simulink model "GS_model"  (R2018b)
settings: Solver=ode5  StartTime=0.0  StopTime=SimuStopTime  FixedStep=T_Simu  RelTol=1e-3
InitFcn:
  | Initial
undefined symbols (not defined in the file or in its folder): Aba10, Aba20, aeroCIP2006_S, aeroCIP2006_X, aeroCIP2006_Y, Agl0, Ass_kS, Ass_n1, Ass_n2, Ass_n3, Ass_n4, Ass_Noise, Ass_R, Ass_Resolution, Ass_TmOrder, AssA_Fix_Abs, AssB_Fix_Abs, AssC_Fix_Abs, AssD_Fix_Abs, AssE_Fix_Aps, AssF_Fix_Aps, C, c_max, c_min, Cd, CenterOfFigNX, CenterOfFigNY, CenterOfFigNZ, CenterOfFigP1, CenterOfFigP2, CenterOfFigPX, CenterOfFigPY, CenterOfFigPZ, Cmu, Crou, DEG2RAD, DiscIntNeverNeededParam, Eg_Dir, Eg_F, Eg_PrepareTime, Eg_r_L_L, Fw_Abf, Fw_Hmax, Fw_J, Fw_Spd0, Fw_Tmax, git_hash_BaseLine, git_hash_Project, Gnss_Noise_Pos, Gnss_Noise_Vel, Gnss_PropgationTime, GyroA_Fix_Abg, GyroA_Noise, GyroB_Fix_Abg, GyroB_Noise, GyroC_Fix_Abg, GyroC_Noise, GyroD_Fix_Abg, GyroD_Noise, h ... (+94)
libraries: simulink x308, sharedutil x46, aerolibutil x37, sharedtransform x31, vrlib x14, aerolibgravity2 x2
(part 16 of 20)

== system GS_model/Subsystem2/Subsystem/Sensor/Magnetometer/MmModel2/Mm_ErrSet/MmErrSet/MmErrSet_Wave ==
  Mm_in : Inport
  ErrSet : Inport  Port=2
  Constant1 : Constant  Value=2
  Constant2 : Constant  Value=3
  Constant3 : Constant
  Demux : Demux  Outputs=3
  MmAxisXErrSet_Wave : Subsystem
  MmAxisXErrSet_Wave1 : Subsystem
  MmAxisXErrSet_Wave2 : Subsystem
  Mux : Mux  Inputs=3
  WaveSet : SignalGenerator  WaveForm=square  Amplitude=0.2
  Mm_out : Outport
  wires:
  Demux/3 -> MmAxisXErrSet_Wave2/1(MmAxis_in)
  Demux/2 -> MmAxisXErrSet_Wave1/1(MmAxis_in)
  Constant2/1 -> MmAxisXErrSet_Wave2/3(MmAxis_Num)
  Constant1/1 -> MmAxisXErrSet_Wave1/3(MmAxis_Num)
  MmAxisXErrSet_Wave2/1(MmAxis_out) -> Mux/3
  MmAxisXErrSet_Wave/1(MmAxis_out) -> Mux/1
  MmAxisXErrSet_Wave1/1(MmAxis_out) -> Mux/2
  WaveSet/1 -> MmAxisXErrSet_Wave/4(MmAxis_WaveSet), MmAxisXErrSet_Wave1/4(MmAxis_WaveSet), MmAxisXErrSet_Wave2/4(MmAxis_WaveSet)
  Constant3/1 -> MmAxisXErrSet_Wave/3(MmAxis_Num)
  ErrSet/1 -> MmAxisXErrSet_Wave/2(ErrSet), MmAxisXErrSet_Wave1/2(ErrSet), MmAxisXErrSet_Wave2/2(ErrSet)
  Demux/1 -> MmAxisXErrSet_Wave/1(MmAxis_in)
  Mux/1 -> Mm_out/1
  Mm_in/1 -> Demux/1

== system GS_model/Subsystem2/Subsystem/Sensor/Magnetometer/MmModel2/Mm_ErrSet/MmErrSet/MmErrSet_WildValue ==
  Mm_in : Inport
  ErrSwitch : Inport  Port=2
  Constant : Constant
  Constant1 : Constant  Value=2
  Constant2 : Constant  Value=3
  Demux : Demux  Outputs=3
  MmAxisXErrSet_WildValue : Subsystem
  MmAxisXErrSet_WildValue1 : Subsystem
  MmAxisXErrSet_WildValue2 : Subsystem
  Mux : Mux  Inputs=3
  WildValue : Constant  Value=2
  Mm_out : Outport
  wires:
  MmAxisXErrSet_WildValue2/1(MmAxis_out) -> Mux/3
  MmAxisXErrSet_WildValue1/1(MmAxis_out) -> Mux/2
  Demux/3 -> MmAxisXErrSet_WildValue2/1(MmAxis_in)
  Demux/2 -> MmAxisXErrSet_WildValue1/1(MmAxis_in)
  Constant2/1 -> MmAxisXErrSet_WildValue2/3(MmAxis_Num)
  Constant1/1 -> MmAxisXErrSet_WildValue1/3(MmAxis_Num)
  MmAxisXErrSet_WildValue/1(MmAxis_out) -> Mux/1
  ErrSwitch/1 -> MmAxisXErrSet_WildValue/2(ErrSwitch), MmAxisXErrSet_WildValue1/2(ErrSwitch), MmAxisXErrSet_WildValue2/2(ErrSwitch)
  Demux/1 -> MmAxisXErrSet_WildValue/1(MmAxis_in)
  WildValue/1 -> MmAxisXErrSet_WildValue/4(MmAxis_WildValue), MmAxisXErrSet_WildValue1/4(MmAxis_WildValue), MmAxisXErrSet_WildValue2/4(MmAxis_WildValue)
  Constant/1 -> MmAxisXErrSet_WildValue/3(MmAxis_Num)
  Mm_in/1 -> Demux/1
  Mux/1 -> Mm_out/1

== system GS_model/Subsystem2/Subsystem/Sensor/Magnetometer/MmModel3/Mm_ErrSet/MmErrSet/MmErrSet_Constant ==
  Mm_in : Inport
  ErrSwitch : Inport  Port=2
  Constant1 : Constant  Value=2
  Constant2 : Constant  Value=3
  Constant3 : Constant
  Demux : Demux  Outputs=3
  MmAxisXErrSet_Constant : Subsystem
  MmAxisXErrSet_Constant1 : Subsystem
  MmAxisXErrSet_Constant2 : Subsystem
  Mux : Mux  Inputs=3
  Mm_out : Outport
  wires:
  Mm_in/1 -> Demux/1
  Mux/1 -> Mm_out/1
  Demux/1 -> MmAxisXErrSet_Constant/1(MmAxis_in)
  ErrSwitch/1 -> MmAxisXErrSet_Constant2/2(ErrSwitch), MmAxisXErrSet_Constant1/2(ErrSwitch), MmAxisXErrSet_Constant/2(ErrSwitch)
  Constant3/1 -> MmAxisXErrSet_Constant/3(MmAxis_Num)
  MmAxisXErrSet_Constant/1(MmAxis_out) -> Mux/1
  Constant1/1 -> MmAxisXErrSet_Constant1/3(MmAxis_Num)
  Constant2/1 -> MmAxisXErrSet_Constant2/3(MmAxis_Num)
  Demux/2 -> MmAxisXErrSet_Constant1/1(MmAxis_in)
  Demux/3 -> MmAxisXErrSet_Constant2/1(MmAxis_in)
  MmAxisXErrSet_Constant1/1(MmAxis_out) -> Mux/2
  MmAxisXErrSet_Constant2/1(MmAxis_out) -> Mux/3

== system GS_model/Subsystem2/Subsystem/Sensor/Magnetometer/MmModel3/Mm_ErrSet/MmErrSet/MmErrSet_Jump ==
  Mm_in : Inport
  ErrSet : Inport  Port=2
  Constant3 : Constant
  Constant4 : Constant  Value=2
  Constant5 : Constant  Value=3
  Demux : Demux  Outputs=3
  JumpSet : Constant  Value=0.2
  MmAxisXErrSet_Jump : Subsystem
  MmAxisXErrSet_Jump1 : Subsystem
  MmAxisXErrSet_Jump2 : Subsystem
  Mux : Mux  Inputs=3
  Mm_out : Outport
  wires:
  Mux/1 -> Mm_out/1
  Mm_in/1 -> Demux/1
  Demux/1 -> MmAxisXErrSet_Jump/1(MmAxis_in)
  ErrSet/1 -> MmAxisXErrSet_Jump2/2(ErrSet), MmAxisXErrSet_Jump1/2(ErrSet), MmAxisXErrSet_Jump/2(ErrSet)
  Constant3/1 -> MmAxisXErrSet_Jump/3(MmAxis_Num)
  JumpSet/1 -> MmAxisXErrSet_Jump2/4(MmAxis_JumpSet), MmAxisXErrSet_Jump1/4(MmAxis_JumpSet), MmAxisXErrSet_Jump/4(MmAxis_JumpSet)
  Constant4/1 -> MmAxisXErrSet_Jump1/3(MmAxis_Num)
  Constant5/1 -> MmAxisXErrSet_Jump2/3(MmAxis_Num)
  Demux/2 -> MmAxisXErrSet_Jump1/1(MmAxis_in)
  Demux/3 -> MmAxisXErrSet_Jump2/1(MmAxis_in)
  MmAxisXErrSet_Jump1/1(MmAxis_out) -> Mux/2
  MmAxisXErrSet_Jump/1(MmAxis_out) -> Mux/1
  MmAxisXErrSet_Jump2/1(MmAxis_out) -> Mux/3

== system GS_model/Subsystem2/Subsystem/Sensor/Magnetometer/MmModel3/Mm_ErrSet/MmErrSet/MmErrSet_Wave ==
  Mm_in : Inport
  ErrSet : Inport  Port=2
  Constant1 : Constant  Value=2
  Constant2 : Constant  Value=3
  Constant3 : Constant
  Demux : Demux  Outputs=3
  MmAxisXErrSet_Wave : Subsystem
  MmAxisXErrSet_Wave1 : Subsystem
  MmAxisXErrSet_Wave2 : Subsystem
  Mux : Mux  Inputs=3
  WaveSet : SignalGenerator  WaveForm=square  Amplitude=0.2
  Mm_out : Outport
  wires:
  Mm_in/1 -> Demux/1
  Mux/1 -> Mm_out/1
  Demux/1 -> MmAxisXErrSet_Wave/1(MmAxis_in)
  ErrSet/1 -> MmAxisXErrSet_Wave2/2(ErrSet), MmAxisXErrSet_Wave1/2(ErrSet), MmAxisXErrSet_Wave/2(ErrSet)
  Constant3/1 -> MmAxisXErrSet_Wave/3(MmAxis_Num)
  WaveSet/1 -> MmAxisXErrSet_Wave2/4(MmAxis_WaveSet), MmAxisXErrSet_Wave1/4(MmAxis_WaveSet), MmAxisXErrSet_Wave/4(MmAxis_WaveSet)
  MmAxisXErrSet_Wave1/1(MmAxis_out) -> Mux/2
  MmAxisXErrSet_Wave/1(MmAxis_out) -> Mux/1
  MmAxisXErrSet_Wave2/1(MmAxis_out) -> Mux/3
  Constant1/1 -> MmAxisXErrSet_Wave1/3(MmAxis_Num)
  Constant2/1 -> MmAxisXErrSet_Wave2/3(MmAxis_Num)
  Demux/2 -> MmAxisXErrSet_Wave1/1(MmAxis_in)
  Demux/3 -> MmAxisXErrSet_Wave2/1(MmAxis_in)

== system GS_model/Subsystem2/Subsystem/Sensor/Magnetometer/MmModel3/Mm_ErrSet/MmErrSet/MmErrSet_WildValue ==
  Mm_in : Inport
  ErrSwitch : Inport  Port=2
  Constant : Constant
  Constant1 : Constant  Value=2
  Constant2 : Constant  Value=3
  Demux : Demux  Outputs=3
  MmAxisXErrSet_WildValue : Subsystem
  MmAxisXErrSet_WildValue1 : Subsystem
  MmAxisXErrSet_WildValue2 : Subsystem
  Mux : Mux  Inputs=3
  WildValue : Constant  Value=2
  Mm_out : Outport
  wires:
  Mux/1 -> Mm_out/1
  Mm_in/1 -> Demux/1
  Constant/1 -> MmAxisXErrSet_WildValue/3(MmAxis_Num)
  WildValue/1 -> MmAxisXErrSet_WildValue2/4(MmAxis_WildValue), MmAxisXErrSet_WildValue1/4(MmAxis_WildValue), MmAxisXErrSet_WildValue/4(MmAxis_WildValue)
  Demux/1 -> MmAxisXErrSet_WildValue/1(MmAxis_in)
  ErrSwitch/1 -> MmAxisXErrSet_WildValue2/2(ErrSwitch), MmAxisXErrSet_WildValue1/2(ErrSwitch), MmAxisXErrSet_WildValue/2(ErrSwitch)
  MmAxisXErrSet_WildValue/1(MmAxis_out) -> Mux/1
  Constant1/1 -> MmAxisXErrSet_WildValue1/3(MmAxis_Num)
  Constant2/1 -> MmAxisXErrSet_WildValue2/3(MmAxis_Num)
  Demux/2 -> MmAxisXErrSet_WildValue1/1(MmAxis_in)
  Demux/3 -> MmAxisXErrSet_WildValue2/1(MmAxis_in)
  MmAxisXErrSet_WildValue1/1(MmAxis_out) -> Mux/2
  MmAxisXErrSet_WildValue2/1(MmAxis_out) -> Mux/3

== system GS_model/Subsystem2/Subsystem/Sensor/Magnetometer/MmModel4/Mm_ErrSet/MmErrSet/MmErrSet_Constant ==
  Mm_in : Inport
  ErrSwitch : Inport  Port=2
  Constant1 : Constant  Value=2
  Constant2 : Constant  Value=3
  Constant3 : Constant
  Demux : Demux  Outputs=3
  MmAxisXErrSet_Constant : Subsystem
  MmAxisXErrSet_Constant1 : Subsystem
  MmAxisXErrSet_Constant2 : Subsystem
  Mux : Mux  Inputs=3
  Mm_out : Outport
  wires:
  MmAxisXErrSet_Constant2/1(MmAxis_out) -> Mux/3
  MmAxisXErrSet_Constant1/1(MmAxis_out) -> Mux/2
  Demux/3 -> MmAxisXErrSet_Constant2/1(MmAxis_in)
  Demux/2 -> MmAxisXErrSet_Constant1/1(MmAxis_in)
  Constant2/1 -> MmAxisXErrSet_Constant2/3(MmAxis_Num)
  Constant1/1 -> MmAxisXErrSet_Constant1/3(MmAxis_Num)
  MmAxisXErrSet_Constant/1(MmAxis_out) -> Mux/1
  Constant3/1 -> MmAxisXErrSet_Constant/3(MmAxis_Num)
  ErrSwitch/1 -> MmAxisXErrSet_Constant/2(ErrSwitch), MmAxisXErrSet_Constant1/2(ErrSwitch), MmAxisXErrSet_Constant2/2(ErrSwitch)
  Demux/1 -> MmAxisXErrSet_Constant/1(MmAxis_in)
  Mux/1 -> Mm_out/1
  Mm_in/1 -> Demux/1

== system GS_model/Subsystem2/Subsystem/Sensor/Magnetometer/MmModel4/Mm_ErrSet/MmErrSet/MmErrSet_Jump ==
  Mm_in : Inport
  ErrSet : Inport  Port=2
  Constant3 : Constant
  Constant4 : Constant  Value=2
  Constant5 : Constant  Value=3
  Demux : Demux  Outputs=3
  JumpSet : Constant  Value=0.2
  MmAxisXErrSet_Jump : Subsystem
  MmAxisXErrSet_Jump1 : Subsystem
  MmAxisXErrSet_Jump2 : Subsystem
  Mux : Mux  Inputs=3
  Mm_out : Outport
  wires:
  MmAxisXErrSet_Jump2/1(MmAxis_out) -> Mux/3
  MmAxisXErrSet_Jump/1(MmAxis_out) -> Mux/1
  MmAxisXErrSet_Jump1/1(MmAxis_out) -> Mux/2
  Demux/3 -> MmAxisXErrSet_Jump2/1(MmAxis_in)
  Demux/2 -> MmAxisXErrSet_Jump1/1(MmAxis_in)
  Constant5/1 -> MmAxisXErrSet_Jump2/3(MmAxis_Num)
  Constant4/1 -> MmAxisXErrSet_Jump1/3(MmAxis_Num)
  JumpSet/1 -> MmAxisXErrSet_Jump/4(MmAxis_JumpSet), MmAxisXErrSet_Jump1/4(MmAxis_JumpSet), MmAxisXErrSet_Jump2/4(MmAxis_JumpSet)
  Constant3/1 -> MmAxisXErrSet_Jump/3(MmAxis_Num)
  ErrSet/1 -> MmAxisXErrSet_Jump/2(ErrSet), MmAxisXErrSet_Jump1/2(ErrSet), MmAxisXErrSet_Jump2/2(ErrSet)
  Demux/1 -> MmAxisXErrSet_Jump/1(MmAxis_in)
  Mm_in/1 -> Demux/1
  Mux/1 -> Mm_out/1

== system GS_model/Subsystem2/Subsystem/Sensor/Magnetometer/MmModel4/Mm_ErrSet/MmErrSet/MmErrSet_Wave ==
  Mm_in : Inport
  ErrSet : Inport  Port=2
  Constant1 : Constant  Value=2
  Constant2 : Constant  Value=3
  Constant3 : Constant
  Demux : Demux  Outputs=3
  MmAxisXErrSet_Wave : Subsystem
  MmAxisXErrSet_Wave1 : Subsystem
  MmAxisXErrSet_Wave2 : Subsystem
  Mux : Mux  Inputs=3
  WaveSet : SignalGenerator  WaveForm=square  Amplitude=0.2
  Mm_out : Outport
  wires:
  Demux/3 -> MmAxisXErrSet_Wave2/1(MmAxis_in)
  Demux/2 -> MmAxisXErrSet_Wave1/1(MmAxis_in)
  Constant2/1 -> MmAxisXErrSet_Wave2/3(MmAxis_Num)
  Constant1/1 -> MmAxisXErrSet_Wave1/3(MmAxis_Num)
  MmAxisXErrSet_Wave2/1(MmAxis_out) -> Mux/3
  MmAxisXErrSet_Wave/1(MmAxis_out) -> Mux/1
  MmAxisXErrSet_Wave1/1(MmAxis_out) -> Mux/2
  WaveSet/1 -> MmAxisXErrSet_Wave/4(MmAxis_WaveSet), MmAxisXErrSet_Wave1/4(MmAxis_WaveSet), MmAxisXErrSet_Wave2/4(MmAxis_WaveSet)
  Constant3/1 -> MmAxisXErrSet_Wave/3(MmAxis_Num)
  ErrSet/1 -> MmAxisXErrSet_Wave/2(ErrSet), MmAxisXErrSet_Wave1/2(ErrSet), MmAxisXErrSet_Wave2/2(ErrSet)
  Demux/1 -> MmAxisXErrSet_Wave/1(MmAxis_in)
  Mux/1 -> Mm_out/1
  Mm_in/1 -> Demux/1

== system GS_model/Subsystem2/Subsystem/Sensor/Magnetometer/MmModel4/Mm_ErrSet/MmErrSet/MmErrSet_WildValue ==
  Mm_in : Inport
  ErrSwitch : Inport  Port=2
  Constant : Constant
  Constant1 : Constant  Value=2
  Constant2 : Constant  Value=3
  Demux : Demux  Outputs=3
  MmAxisXErrSet_WildValue : Subsystem
  MmAxisXErrSet_WildValue1 : Subsystem
  MmAxisXErrSet_WildValue2 : Subsystem
  Mux : Mux  Inputs=3
  WildValue : Constant  Value=2
  Mm_out : Outport
  wires:
  MmAxisXErrSet_WildValue2/1(MmAxis_out) -> Mux/3
  MmAxisXErrSet_WildValue1/1(MmAxis_out) -> Mux/2
  Demux/3 -> MmAxisXErrSet_WildValue2/1(MmAxis_in)
  Demux/2 -> MmAxisXErrSet_WildValue1/1(MmAxis_in)
  Constant2/1 -> MmAxisXErrSet_WildValue2/3(MmAxis_Num)
  Constant1/1 -> MmAxisXErrSet_WildValue1/3(MmAxis_Num)
  MmAxisXErrSet_WildValue/1(MmAxis_out) -> Mux/1
  ErrSwitch/1 -> MmAxisXErrSet_WildValue/2(ErrSwitch), MmAxisXErrSet_WildValue1/2(ErrSwitch), MmAxisXErrSet_WildValue2/2(ErrSwitch)
  Demux/1 -> MmAxisXErrSet_WildValue/1(MmAxis_in)
  WildValue/1 -> MmAxisXErrSet_WildValue/4(MmAxis_WildValue), MmAxisXErrSet_WildValue1/4(MmAxis_WildValue), MmAxisXErrSet_WildValue2/4(MmAxis_WildValue)
  Constant/1 -> MmAxisXErrSet_WildValue/3(MmAxis_Num)
  Mm_in/1 -> Demux/1
  Mux/1 -> Mm_out/1

== system GS_model/Subsystem2/Subsystem/Sensor/StA&B&C&DModel1/StAMathModel/StErrSet/StAErrSet/AssErrSet_WildValue ==
  Qin : Inport
  ErrValue : Inport  Port=2
  ErrSwitch : Inport  Port=3
  Product : Product
  Switch2 : Switch  Criteria=u2 > Threshold  Threshold=0.5
  Q_out : Outport
  wires:
  ErrSwitch/1 -> Switch2/2
  Switch2/1 -> Q_out/1
  Qin/1 -> Product/2, Switch2/3
  ErrValue/1 -> Product/1
  Product/1 -> Switch2/1

== system GS_model/Subsystem2/Subsystem/Sensor/StA&B&C&DModel1/StAMathModel/StErrSet/StAErrSet/StErrSet_Constant ==
  Q_in : Inport
  ErrSwitch : Inport  Port=2
  Memory : Memory  InitialCondition=[1;0;0;0]
  Switch1 : Switch  Criteria=u2 > Threshold  Threshold=0.5
  Q_out : Outport
  wires:
  Q_in/1 -> Switch1/3
  Switch1/1 -> Memory/1, Q_out/1
  Memory/1 -> Switch1/1
  ErrSwitch/1 -> Switch1/2

== system GS_model/Subsystem2/Subsystem/Sensor/StA&B&C&DModel1/StAMathModel/StErrSet/StAErrSet/StErrSet_Jump ==
  Qin : Inport
  ErrValue : Inport  Port=2
  ErrSwitch : Inport  Port=3
  StJumpErrAmpCoff : Inport  Port=4
  Product : Product
  Quaternion Multiplication : aerolibutil/Quaternion Multiplication
  Rotation Angles to Quaternions : sharedtransform/Rotation Angles to Quaternions  rotationOrder=XYZ  aMode=aMode
      settings: SourceProductBaseCode=AE,PW,MT,VE,VP
  Switch3 : Switch  Criteria=u2 > Threshold  Threshold=0.5
  Q_out : Outport
  wires:
  Switch3/1 -> Q_out/1
  Qin/1 -> Switch3/3, Quaternion Multiplication/1
  Rotation Angles to Quaternions/1 -> Quaternion Multiplication/2
  Quaternion Multiplication/1 -> Switch3/1
  ErrSwitch/1 -> Switch3/2
  ErrValue/1 -> Product/1
  Product/1 -> Rotation Angles to Quaternions/1
  StJumpErrAmpCoff/1 -> Product/2

== system GS_model/Subsystem2/Subsystem/Sensor/StA&B&C&DModel1/StAMathModel/StErrSet/StAErrSet/StErrSet_Wave ==
  Qin : Inport
  ErrValue : Inport  Port=2
  ErrSwitch : Inport  Port=3
  StWaveErrAmp : Inport  Port=4
  Constant : Constant  Value=0
  Mux : Mux  Inputs=3
  Product : Product
  Quaternion Multiplication : aerolibutil/Quaternion Multiplication
  Rotation Angles to Quaternions : sharedtransform/Rotation Angles to Quaternions  rotationOrder=YXZ  aMode=aMode
      settings: SourceProductBaseCode=AE,PW,MT,VE,VP
  Switch4 : Switch  Criteria=u2 > Threshold  Threshold=0.5
  Q_out : Outport
  wires:
  Switch4/1 -> Q_out/1
  ErrSwitch/1 -> Switch4/2
  ErrValue/1 -> Mux/2
  Mux/1 -> Product/1
  Product/1 -> Rotation Angles to Quaternions/1
  Quaternion Multiplication/1 -> Switch4/1
  Qin/1 -> Switch4/3, Quaternion Multiplication/1
  Rotation Angles to Quaternions/1 -> Quaternion Multiplication/2
  Constant/1 -> Mux/1, Mux/3
  StWaveErrAmp/1 -> Product/2

== system GS_model/Subsystem2/Subsystem/Sensor/StA&B&C&DModel1/StAMathModel1/StErrSet/StAErrSet/AssErrSet_WildValue ==
  Qin : Inport
  ErrValue : Inport  Port=2
  ErrSwitch : Inport  Port=3
  Product : Product
  Switch2 : Switch  Criteria=u2 > Threshold  Threshold=0.5
  Q_out : Outport
  wires:
  Product/1 -> Switch2/1
  ErrValue/1 -> Product/1
  Qin/1 -> Switch2/3, Product/2
  Switch2/1 -> Q_out/1
  ErrSwitch/1 -> Switch2/2

== system GS_model/Subsystem2/Subsystem/Sensor/StA&B&C&DModel1/StAMathModel1/StErrSet/StAErrSet/StErrSet_Constant ==
  Q_in : Inport
  ErrSwitch : Inport  Port=2
  Memory : Memory  InitialCondition=[1;0;0;0]
  Switch1 : Switch  Criteria=u2 > Threshold  Threshold=0.5
  Q_out : Outport
  wires:
  ErrSwitch/1 -> Switch1/2
  Memory/1 -> Switch1/1
  Switch1/1 -> Q_out/1, Memory/1
  Q_in/1 -> Switch1/3

== system GS_model/Subsystem2/Subsystem/Sensor/StA&B&C&DModel1/StAMathModel1/StErrSet/StAErrSet/StErrSet_Jump ==
  Qin : Inport
  ErrValue : Inport  Port=2
  ErrSwitch : Inport  Port=3
  StJumpErrAmpCoff : Inport  Port=4
  Product : Product
  Quaternion Multiplication : aerolibutil/Quaternion Multiplication
  Rotation Angles to Quaternions : sharedtransform/Rotation Angles to Quaternions  rotationOrder=XYZ  aMode=aMode
      settings: SourceProductBaseCode=AE,PW,MT,VE,VP
  Switch3 : Switch  Criteria=u2 > Threshold  Threshold=0.5
  Q_out : Outport
  wires:
  StJumpErrAmpCoff/1 -> Product/2
  Product/1 -> Rotation Angles to Quaternions/1
  ErrValue/1 -> Product/1
  ErrSwitch/1 -> Switch3/2
  Quaternion Multiplication/1 -> Switch3/1
  Rotation Angles to Quaternions/1 -> Quaternion Multiplication/2
  Qin/1 -> Quaternion Multiplication/1, Switch3/3
  Switch3/1 -> Q_out/1

== system GS_model/Subsystem2/Subsystem/Sensor/StA&B&C&DModel1/StAMathModel1/StErrSet/StAErrSet/StErrSet_Wave ==
  Qin : Inport
  ErrValue : Inport  Port=2
  ErrSwitch : Inport  Port=3
  StWaveErrAmp : Inport  Port=4
  Constant : Constant  Value=0
  Mux : Mux  Inputs=3
  Product : Product
  Quaternion Multiplication : aerolibutil/Quaternion Multiplication
  Rotation Angles to Quaternions : sharedtransform/Rotation Angles to Quaternions  rotationOrder=YXZ  aMode=aMode
      settings: SourceProductBaseCode=AE,PW,MT,VE,VP
  Switch4 : Switch  Criteria=u2 > Threshold  Threshold=0.5
  Q_out : Outport
  wires:
  StWaveErrAmp/1 -> Product/2
  Constant/1 -> Mux/3, Mux/1
  Rotation Angles to Quaternions/1 -> Quaternion Multiplication/2
  Qin/1 -> Quaternion Multiplication/1, Switch4/3
  Quaternion Multiplication/1 -> Switch4/1
  Product/1 -> Rotation Angles to Quaternions/1
  Mux/1 -> Product/1
  ErrValue/1 -> Mux/2
  ErrSwitch/1 -> Switch4/2
  Switch4/1 -> Q_out/1

== system GS_model/Subsystem2/Subsystem/Sensor/StA&B&C&DModel1/StAMathModel2/StErrSet/StAErrSet/AssErrSet_WildValue ==
  Qin : Inport
  ErrValue : Inport  Port=2
  ErrSwitch : Inport  Port=3
  Product : Product
  Switch2 : Switch  Criteria=u2 > Threshold  Threshold=0.5
  Q_out : Outport
  wires:
  ErrSwitch/1 -> Switch2/2
  Switch2/1 -> Q_out/1
  Qin/1 -> Product/2, Switch2/3
  ErrValue/1 -> Product/1
  Product/1 -> Switch2/1

== system GS_model/Subsystem2/Subsystem/Sensor/StA&B&C&DModel1/StAMathModel2/StErrSet/StAErrSet/StErrSet_Constant ==
  Q_in : Inport
  ErrSwitch : Inport  Port=2
  Memory : Memory  InitialCondition=[1;0;0;0]
  Switch1 : Switch  Criteria=u2 > Threshold  Threshold=0.5
  Q_out : Outport
  wires:
  Q_in/1 -> Switch1/3
  Switch1/1 -> Memory/1, Q_out/1
  Memory/1 -> Switch1/1
  ErrSwitch/1 -> Switch1/2

== system GS_model/Subsystem2/Subsystem/Sensor/StA&B&C&DModel1/StAMathModel2/StErrSet/StAErrSet/StErrSet_Jump ==
  Qin : Inport
  ErrValue : Inport  Port=2
  ErrSwitch : Inport  Port=3
  StJumpErrAmpCoff : Inport  Port=4
  Product : Product
  Quaternion Multiplication : aerolibutil/Quaternion Multiplication
  Rotation Angles to Quaternions : sharedtransform/Rotation Angles to Quaternions  rotationOrder=XYZ  aMode=aMode
      settings: SourceProductBaseCode=AE,PW,MT,VE,VP
  Switch3 : Switch  Criteria=u2 > Threshold  Threshold=0.5
  Q_out : Outport
  wires:
  Switch3/1 -> Q_out/1
  Qin/1 -> Switch3/3, Quaternion Multiplication/1
  Rotation Angles to Quaternions/1 -> Quaternion Multiplication/2
  Quaternion Multiplication/1 -> Switch3/1
  ErrSwitch/1 -> Switch3/2
  ErrValue/1 -> Product/1
  Product/1 -> Rotation Angles to Quaternions/1
  StJumpErrAmpCoff/1 -> Product/2

== system GS_model/Subsystem2/Subsystem/Sensor/StA&B&C&DModel1/StAMathModel2/StErrSet/StAErrSet/StErrSet_Wave ==
  Qin : Inport
  ErrValue : Inport  Port=2
  ErrSwitch : Inport  Port=3
  StWaveErrAmp : Inport  Port=4
  Constant : Constant  Value=0
  Mux : Mux  Inputs=3
  Product : Product
  Quaternion Multiplication : aerolibutil/Quaternion Multiplication
  Rotation Angles to Quaternions : sharedtransform/Rotation Angles to Quaternions  rotationOrder=YXZ  aMode=aMode
      settings: SourceProductBaseCode=AE,PW,MT,VE,VP
  Switch4 : Switch  Criteria=u2 > Threshold  Threshold=0.5
  Q_out : Outport
  wires:
  Switch4/1 -> Q_out/1
  ErrSwitch/1 -> Switch4/2
  ErrValue/1 -> Mux/2
  Mux/1 -> Product/1
  Product/1 -> Rotation Angles to Quaternions/1
  Quaternion Multiplication/1 -> Switch4/1
  Qin/1 -> Switch4/3, Quaternion Multiplication/1
  Rotation Angles to Quaternions/1 -> Quaternion Multiplication/2
  Constant/1 -> Mux/1, Mux/3
  StWaveErrAmp/1 -> Product/2

== system GS_model/Subsystem2/Subsystem/Sensor/StA&B&C&DModel1/StAMathModel3/StErrSet/StAErrSet/AssErrSet_WildValue ==
  Qin : Inport
  ErrValue : Inport  Port=2
  ErrSwitch : Inport  Port=3
  Product : Product
  Switch2 : Switch  Criteria=u2 > Threshold  Threshold=0.5
  Q_out : Outport
  wires:
  Product/1 -> Switch2/1
  ErrValue/1 -> Product/1
  Qin/1 -> Switch2/3, Product/2
  Switch2/1 -> Q_out/1
  ErrSwitch/1 -> Switch2/2

== system GS_model/Subsystem2/Subsystem/Sensor/StA&B&C&DModel1/StAMathModel3/StErrSet/StAErrSet/StErrSet_Constant ==
  Q_in : Inport
  ErrSwitch : Inport  Port=2
  Memory : Memory  InitialCondition=[1;0;0;0]
  Switch1 : Switch  Criteria=u2 > Threshold  Threshold=0.5
  Q_out : Outport
  wires:
  ErrSwitch/1 -> Switch1/2
  Memory/1 -> Switch1/1
  Switch1/1 -> Q_out/1, Memory/1
  Q_in/1 -> Switch1/3

== system GS_model/Subsystem2/Subsystem/Sensor/StA&B&C&DModel1/StAMathModel3/StErrSet/StAErrSet/StErrSet_Jump ==
  Qin : Inport
  ErrValue : Inport  Port=2
  ErrSwitch : Inport  Port=3
  StJumpErrAmpCoff : Inport  Port=4
  Product : Product
  Quaternion Multiplication : aerolibutil/Quaternion Multiplication
  Rotation Angles to Quaternions : sharedtransform/Rotation Angles to Quaternions  rotationOrder=XYZ  aMode=aMode
      settings: SourceProductBaseCode=AE,PW,MT,VE,VP
  Switch3 : Switch  Criteria=u2 > Threshold  Threshold=0.5
  Q_out : Outport
  wires:
  StJumpErrAmpCoff/1 -> Product/2
  Product/1 -> Rotation Angles to Quaternions/1
  ErrValue/1 -> Product/1
  ErrSwitch/1 -> Switch3/2
  Quaternion Multiplication/1 -> Switch3/1
  Rotation Angles to Quaternions/1 -> Quaternion Multiplication/2
  Qin/1 -> Quaternion Multiplication/1, Switch3/3
  Switch3/1 -> Q_out/1

== system GS_model/Subsystem2/Subsystem/Sensor/StA&B&C&DModel1/StAMathModel3/StErrSet/StAErrSet/StErrSet_Wave ==
  Qin : Inport
  ErrValue : Inport  Port=2
  ErrSwitch : Inport  Port=3
  StWaveErrAmp : Inport  Port=4
  Constant : Constant  Value=0
  Mux : Mux  Inputs=3
  Product : Product
  Quaternion Multiplication : aerolibutil/Quaternion Multiplication
  Rotation Angles to Quaternions : sharedtransform/Rotation Angles to Quaternions  rotationOrder=YXZ  aMode=aMode
      settings: SourceProductBaseCode=AE,PW,MT,VE,VP
  Switch4 : Switch  Criteria=u2 > Threshold  Threshold=0.5
  Q_out : Outport
  wires:
  StWaveErrAmp/1 -> Product/2
  Constant/1 -> Mux/3, Mux/1
  Rotation Angles to Quaternions/1 -> Quaternion Multiplication/2
  Qin/1 -> Quaternion Multiplication/1, Switch4/3
  Quaternion Multiplication/1 -> Switch4/1
  Product/1 -> Rotation Angles to Quaternions/1
  Mux/1 -> Product/1
  ErrValue/1 -> Mux/2
  ErrSwitch/1 -> Switch4/2
  Switch4/1 -> Q_out/1

== system GS_model/Subsystem2/Subsystem/PhysicsModel/Environment/Sun  press torque/Sun  press torque2/Sun  press torque/+Y SunPanel/Compute press of sun radiation ==
  note: Huang zhen gui P67
  note: u_t
  note: u_n
  Sun(p) : Inport
  TC_SunPressCoeff : Inport  Port=2
  1/r : Subsystem  TreatAsAtomicUnit=on
  3x3 Cross Product : sharedutil/3x3 Cross Product  aMode=aMode
      settings: SourceProductBaseCode=AE,PW,MT,VE,VP
  3x3 Cross Product1 : sharedutil/3x3 Cross Product  aMode=aMode
      settings: SourceProductBaseCode=AE,PW,MT,VE,VP
  Board Orientation : Constant  Value=n_P1N  VectorParams1D=off
  Board Orientation1 : Constant  Value=n_P1P  VectorParams1D=off
  Crd2 : Constant  Value=2/3*Crou*Cmu
  Dot Product : DotProduct  InputSameDT=on  OutDataTypeStr=Inherit: Inherit via internal rule
  Dot Product1 : DotProduct  InputSameDT=on  OutDataTypeStr=Inherit: Inherit via internal rule
  Fcn : Fcn  Expr=u(3)
  Gain : Gain  Gain=1+Crou*(1-Cmu)
  Gain1 : Gain  Gain=-1  SaturateOnIntegerOverflow=on  OutDataTypeStr=Inherit: Same as input  ParamDataTypeStr=Inherit: Same as input
  Gain2 : Gain  Gain=SConst/C*S_P1
  Gain4 : Gain  Gain=1-Crou+Crou*Cmu
  Product{1..5} (5 alike) : Product  SaturateOnIntegerOverflow=on  OutDataTypeStr=Inherit: Same as first input
  Sum1 : Sum  SaturateOnIntegerOverflow=on  InputSameDT=on  OutDataTypeStr=Inherit: Same as first input
  Sum2 : Sum  Inputs=|++  SaturateOnIntegerOverflow=on  InputSameDT=on  OutDataTypeStr=Inherit: Same as first input
  Switch2 : Switch  SaturateOnIntegerOverflow=on  InputSameDT=on
  Trigonometric Function1 : Trigonometry
  Trigonometric Function2 : Trigonometry  Operator=acos
  F(p) : Outport
  wires:
  TC_SunPressCoeff/1 -> Product5/2
  Product5/1 -> Product3/2
  Gain2/1 -> Product5/1
  Dot Product1/1 -> 1/r/1(In1)
  Trigonometric Function1/1 -> Gain4/1
  Product1/1 -> Product2/1
  Product4/1 -> Sum1/2
  Product2/1 -> Sum1/1
  Product3/1 -> F(p)/1
  3x3 Cross Product1/1 -> Dot Product1/2, Product1/1, Dot Product1/1
  1/r/1(Out1) -> Product1/2
  3x3 Cross Product/1 -> 3x3 Cross Product1/1
  Gain4/1 -> Product2/2
  Trigonometric Function2/1 -> Trigonometric Function1/1
  Sun(p)/1 -> 3x3 Cross Product/1, Dot Product/1, Fcn/1
  Dot Product/1 -> Gain2/1, Gain/1, Trigonometric Function2/1
  Sum1/1 -> Product3/1
  Switch2/1 -> Dot Product/2, Gain1/1, 3x3 Cross Product1/2, 3x3 Cross Product/2
  Gain1/1 -> Product4/2
  Crd2/1 -> Sum2/2
  Sum2/1 -> Product4/1
  Gain/1 -> Sum2/1
  Fcn/1 -> Switch2/2
  Board Orientation/1 -> Switch2/3
  Board Orientation1/1 -> Switch2/1

== system GS_model/Subsystem2/Subsystem/PhysicsModel/Environment/Sun  press torque/Sun  press torque2/Sun  press torque/+Y SunPanel/compute centroi 1 ==
  Cent : Inport
  Abp_PY : Inport  Port=2
  Aba1 : Constant  Value=Aba10  VectorParams1D=off
  Product1 : Product  Multiplication=Matrix(*)  SaturateOnIntegerOverflow=on  InputSameDT=on  OutDataTypeStr=Inherit: Same as first input
  Product12 : Product  Multiplication=Matrix(*)  SaturateOnIntegerOverflow=on  InputSameDT=on  OutDataTypeStr=Inherit: Same as first input
  Sum2 : Sum  Inputs=|+-
  Sum3 : Sum  Inputs=+++  SaturateOnIntegerOverflow=on  InputSameDT=on  OutDataTypeStr=Inherit: Same as first input
  y3 : Constant  Value=CenterOfFigP1  VectorParams1D=off
  ·«°åa°²×°µãÎ»ÖÃ(L) : Constant  Value=r_L_a1_b  VectorParams1D=off
  ·«°åp°²×°µãÎ»ÖÃ(a0) : Constant  Value=r_a1_p1_a1  VectorParams1D=off
  r : Outport
  wires:
  Product12/1 -> Sum3/1
  Aba1/1 -> Product1/1
  ·«°åp°²×°µãÎ»ÖÃ(a0)/1 -> Product1/2
  Product1/1 -> Sum3/2
  y3/1 -> Product12/2
  ·«°åa°²×°µãÎ»ÖÃ(L)/1 -> Sum3/3
  Sum3/1 -> Sum2/1
  Abp_PY/1 -> Product12/1
  Cent/1 -> Sum2/2
  Sum2/1 -> r/1

== system GS_model/Subsystem2/Subsystem/PhysicsModel/Environment/Sun  press torque/Sun  press torque2/Sun  press torque/-Y SunPanel/Compute press of sun radiation ==
  note: u_n
  note: u_t
  note: Huang zhen gui P67
  Sun(p) : Inport
  TC_SunPressCoeff : Inport  Port=2
  1/r : Subsystem  TreatAsAtomicUnit=on
  3x3 Cross Product : sharedutil/3x3 Cross Product  aMode=aMode
      settings: SourceProductBaseCode=AE,PW,MT,VE,VP
  3x3 Cross Product1 : sharedutil/3x3 Cross Product  aMode=aMode
      settings: SourceProductBaseCode=AE,PW,MT,VE,VP
  Board Orientation : Constant  Value=n_P2N  VectorParams1D=off
  Board Orientation1 : Constant  Value=n_P2P  VectorParams1D=off
  Crd2 : Constant  Value=2/3*Crou*Cmu
  Dot Product : DotProduct  InputSameDT=on  OutDataTypeStr=Inherit: Inherit via internal rule
  Dot Product1 : DotProduct  InputSameDT=on  OutDataTypeStr=Inherit: Inherit via internal rule
  Fcn : Fcn  Expr=u(3)
  Gain : Gain  Gain=1+Crou*(1-Cmu)
  Gain1 : Gain  Gain=-1  SaturateOnIntegerOverflow=on  OutDataTypeStr=Inherit: Same as input  ParamDataTypeStr=Inherit: Same as input
  Gain2 : Gain  Gain=SConst/C*S_P2
  Gain4 : Gain  Gain=1-Crou+Crou*Cmu
  Product{1..5} (5 alike) : Product  SaturateOnIntegerOverflow=on  OutDataTypeStr=Inherit: Same as first input
  Sum1 : Sum  SaturateOnIntegerOverflow=on  InputSameDT=on  OutDataTypeStr=Inherit: Same as first input
  Sum2 : Sum  Inputs=|++  SaturateOnIntegerOverflow=on  InputSameDT=on  OutDataTypeStr=Inherit: Same as first input
  Switch2 : Switch  SaturateOnIntegerOverflow=on  InputSameDT=on
  Trigonometric Function1 : Trigonometry
  Trigonometric Function2 : Trigonometry  Operator=acos
  F(p) : Outport
  wires:
  Board Orientation1/1 -> Switch2/1
  Board Orientation/1 -> Switch2/3
  Fcn/1 -> Switch2/2
  Gain/1 -> Sum2/1
  Sum2/1 -> Product4/1
  Crd2/1 -> Sum2/2
  Gain1/1 -> Product4/2
  Switch2/1 -> Dot Product/2, Gain1/1, 3x3 Cross Product1/2, 3x3 Cross Product/2
  Sum1/1 -> Product3/1
  Dot Product/1 -> Gain2/1, Gain/1, Trigonometric Function2/1
  Sun(p)/1 -> Fcn/1, 3x3 Cross Product/1, Dot Product/1
  Trigonometric Function2/1 -> Trigonometric Function1/1
  Gain4/1 -> Product2/2
  3x3 Cross Product/1 -> 3x3 Cross Product1/1
  1/r/1(Out1) -> Product1/2
  3x3 Cross Product1/1 -> Dot Product1/1, Product1/1, Dot Product1/2
  Product3/1 -> F(p)/1
  Product2/1 -> Sum1/1
  Product4/1 -> Sum1/2
  Product1/1 -> Product2/1
  Trigonometric Function1/1 -> Gain4/1
  Dot Product1/1 -> 1/r/1(In1)
  Gain2/1 -> Product5/1
  Product5/1 -> Product3/2
  TC_SunPressCoeff/1 -> Product5/2

== system GS_model/Subsystem2/Subsystem/PhysicsModel/Environment/Sun  press torque/Sun  press torque2/Sun  press torque/-Y SunPanel/compute centroi 1 ==
  Cent : Inport
  Abp_NY : Inport  Port=2
  Aba1 : Constant  Value=Aba20  VectorParams1D=off
  Product1 : Product  Multiplication=Matrix(*)  SaturateOnIntegerOverflow=on  InputSameDT=on  OutDataTypeStr=Inherit: Same as first input
  Product12 : Product  Multiplication=Matrix(*)  SaturateOnIntegerOverflow=on  InputSameDT=on  OutDataTypeStr=Inherit: Same as first input
  Sum2 : Sum  Inputs=|+-
  Sum3 : Sum  Inputs=+++  SaturateOnIntegerOverflow=on  InputSameDT=on  OutDataTypeStr=Inherit: Same as first input
  y3 : Constant  Value=CenterOfFigP2  VectorParams1D=off
  ·«°åa°²×°µãÎ»ÖÃ(L) : Constant  Value=r_L_a2_b  VectorParams1D=off
  ·«°åp°²×°µãÎ»ÖÃ(a0) : Constant  Value=r_a2_p2_a2  VectorParams1D=off
  r : Outport
  wires:
  Sum2/1 -> r/1
  Cent/1 -> Sum2/2
  Abp_NY/1 -> Product12/1
  Sum3/1 -> Sum2/1
  ·«°åa°²×°µãÎ»ÖÃ(L)/1 -> Sum3/3
  y3/1 -> Product12/2
  Product1/1 -> Sum3/2
  ·«°åp°²×°µãÎ»ÖÃ(a0)/1 -> Product1/2
  Aba1/1 -> Product1/1
  Product12/1 -> Sum3/1

== system GS_model/Subsystem2/Subsystem/PhysicsModel/Environment/Sun  press torque/Sun  press torque2/Sun  press torque/Torque from   satalite board/Torque from  board perpendicular to z axis  ==
  Sun Orientation : Inport
  Cent : Inport  Port=2
  TC_SunPressCoeff : Inport  Port=3
  3x3 Cross Product : sharedutil/3x3 Cross Product  aMode=aMode
      settings: SourceProductBaseCode=AE,PW,MT,VE,VP
  Compute press of sun radiation : Subsystem  TreatAsAtomicUnit=on
  compute centroi 1 : Subsystem  TreatAsAtomicUnit=on
  Tz : Outport
  Fz : Outport  Port=2
  wires:
  compute centroi 1/1(r_z) -> 3x3 Cross Product/1
  Sun Orientation/1 -> compute centroi 1/1(Orientation), Compute press of sun radiation/1(Sun Orientation)
  3x3 Cross Product/1 -> Tz/1
  Compute press of sun radiation/1(Fz) -> 3x3 Cross Product/2, Fz/1
  Cent/1 -> compute centroi 1/2(Cent)
  TC_SunPressCoeff/1 -> Compute press of sun radiation/2(TC_SunPressCoeff)

== system GS_model/Subsystem2/Subsystem/PhysicsModel/Environment/Sun  press torque/Sun  press torque2/Sun  press torque/Torque from   satalite board/Torque from board perpendicular to x axis ==
  Sun Orientation : Inport
  Cent : Inport  Port=2
  TC_SunPressCoeff : Inport  Port=3
  3x3 Cross Product : sharedutil/3x3 Cross Product  aMode=aMode
      settings: SourceProductBaseCode=AE,PW,MT,VE,VP
  Compute press of sun radiation : Subsystem  TreatAsAtomicUnit=on
  compute centroi 1 : Subsystem  TreatAsAtomicUnit=on
  Tx : Outport
  Fx : Outport  Port=2
  wires:
  compute centroi 1/1(r_x) -> 3x3 Cross Product/1
  Sun Orientation/1 -> compute centroi 1/1(Orientation), Compute press of sun radiation/1(Sun Orientation)
  3x3 Cross Product/1 -> Tx/1
  Compute press of sun radiation/1(Fx) -> 3x3 Cross Product/2, Fx/1
  Cent/1 -> compute centroi 1/2(Cent)
  TC_SunPressCoeff/1 -> Compute press of sun radiation/2(TC_SunPressCoeff)

== system GS_model/Subsystem2/Subsystem/PhysicsModel/Environment/Sun  press torque/Sun  press torque2/Sun  press torque/Torque from   satalite board/Torque from board perpendicular to y axis ==
  Sun Orientation : Inport
  Cent : Inport  Port=2
  TC_SunPressCoeff : Inport  Port=3
  3x3 Cross Product : sharedutil/3x3 Cross Product  aMode=aMode
      settings: SourceProductBaseCode=AE,PW,MT,VE,VP
  Compute press of sun radiation1 : Subsystem  TreatAsAtomicUnit=on
  compute centroi 1 : Subsystem  TreatAsAtomicUnit=on
  Ty : Outport
  Fy : Outport  Port=2
  wires:
  compute centroi 1/1(r_y) -> 3x3 Cross Product/1
  Sun Orientation/1 -> Compute press of sun radiation1/1(Sun Orientation), compute centroi 1/1(Orientation)
  3x3 Cross Product/1 -> Ty/1
  Compute press of sun radiation1/1(Fy) -> 3x3 Cross Product/2, Fy/1
  Cent/1 -> compute centroi 1/2(Cent)
  TC_SunPressCoeff/1 -> Compute press of sun radiation1/2(TC_SunPressCoeff)

== system GS_model/Subsystem2/Subsystem/Sensor/Ass/BodyAss(A&B&C&D)Model/Subsystem/AssErrModel/AssErrSet/AssErrSet_Constant ==
  ErrSwitch : Inport
  Ass_in : Inport  Port=2
  Memory : Memory  InitialCondition=[0;0;0;0]
  Switch1 : Switch  Criteria=u2 > Threshold  Threshold=0.5
  Ass_out : Outport
  wires:
  Switch1/1 -> Ass_out/1, Memory/1
  Memory/1 -> Switch1/1
  Ass_in/1 -> Switch1/3
  ErrSwitch/1 -> Switch1/2

== system GS_model/Subsystem2/Subsystem/Sensor/Ass/BodyAss(A&B&C&D)Model/Subsystem/AssErrModel/AssErrSet/AssErrSet_Jump ==
  Ass_in : Inport
  ErrValue : Inport  Port=2
  ErrSwitch : Inport  Port=3
  AssJumpErrAmpCoff : Inport  Port=4
  Add1 : Sum
  Product1 : Product  SaturateOnIntegerOverflow=on  OutDataTypeStr=Inherit: Same as first input
  Switch3 : Switch  Criteria=u2 > Threshold  Threshold=0.5
  Ass_out : Outport
  wires:
  Switch3/1 -> Ass_out/1
  ErrSwitch/1 -> Switch3/2
  Ass_in/1 -> Add1/2, Switch3/3
  AssJumpErrAmpCoff/1 -> Product1/2
  ErrValue/1 -> Product1/1
  Add1/1 -> Switch3/1
  Product1/1 -> Add1/1

== system GS_model/Subsystem2/Subsystem/Sensor/Ass/BodyAss(A&B&C&D)Model/Subsystem/AssErrModel/AssErrSet/AssErrSet_Wave ==
  Ass_in : Inport
  ErrValue : Inport  Port=2
  ErrSwitch : Inport  Port=3
  AssWaveErrAmpCoff : Inport  Port=4
  Add2 : Sum
  Product2 : Product  SaturateOnIntegerOverflow=on  OutDataTypeStr=Inherit: Same as first input
  Switch4 : Switch  Criteria=u2 > Threshold  Threshold=0.5
  Ass_out : Outport
  wires:
  ErrSwitch/1 -> Switch4/2
  Add2/1 -> Switch4/1
  Switch4/1 -> Ass_out/1
  Ass_in/1 -> Add2/2, Switch4/3
  Product2/1 -> Add2/1
  AssWaveErrAmpCoff/1 -> Product2/2
  ErrValue/1 -> Product2/1

== system GS_model/Subsystem2/Subsystem/Sensor/Ass/BodyAss(A&B&C&D)Model/Subsystem/AssErrModel/AssErrSet/AssErrSet_WildValue ==
  Ass_in : Inport
  ErrValue : Inport  Port=2
  ErrSwitch : Inport  Port=3
  Add : Sum
  Switch2 : Switch  Criteria=u2 > Threshold  Threshold=0.5
  Ass_out : Outport
  wires:
  Add/1 -> Switch2/1
  Ass_in/1 -> Add/2, Switch2/3
  Switch2/1 -> Ass_out/1
  ErrSwitch/1 -> Switch2/2
  ErrValue/1 -> Add/1

== system GS_model/Subsystem2/Subsystem/Sensor/Ass/BodyAss(A&B&C&D)Model/Subsystem1/AssErrModel/AssErrSet/AssErrSet_Constant ==
  ErrSwitch : Inport
  Ass_in : Inport  Port=2
  Memory : Memory  InitialCondition=[0;0;0;0]
  Switch1 : Switch  Criteria=u2 > Threshold  Threshold=0.5
  Ass_out : Outport
  wires:
  ErrSwitch/1 -> Switch1/2
  Ass_in/1 -> Switch1/3
  Memory/1 -> Switch1/1
  Switch1/1 -> Memory/1, Ass_out/1

== system GS_model/Subsystem2/Subsystem/Sensor/Ass/BodyAss(A&B&C&D)Model/Subsystem1/AssErrModel/AssErrSet/AssErrSet_Jump ==
  Ass_in : Inport
  ErrValue : Inport  Port=2
  ErrSwitch : Inport  Port=3
  AssJumpErrAmpCoff : Inport  Port=4
  Add1 : Sum
  Product1 : Product  SaturateOnIntegerOverflow=on  OutDataTypeStr=Inherit: Same as first input
  Switch3 : Switch  Criteria=u2 > Threshold  Threshold=0.5
  Ass_out : Outport
  wires:
  Product1/1 -> Add1/1
  Add1/1 -> Switch3/1
  ErrValue/1 -> Product1/1
  AssJumpErrAmpCoff/1 -> Product1/2
  Ass_in/1 -> Switch3/3, Add1/2
  ErrSwitch/1 -> Switch3/2
  Switch3/1 -> Ass_out/1

== system GS_model/Subsystem2/Subsystem/Sensor/Ass/BodyAss(A&B&C&D)Model/Subsystem1/AssErrModel/AssErrSet/AssErrSet_Wave ==
  Ass_in : Inport
  ErrValue : Inport  Port=2
  ErrSwitch : Inport  Port=3
  AssWaveErrAmpCoff : Inport  Port=4
  Add2 : Sum
  Product2 : Product  SaturateOnIntegerOverflow=on  OutDataTypeStr=Inherit: Same as first input
  Switch4 : Switch  Criteria=u2 > Threshold  Threshold=0.5
  Ass_out : Outport
  wires:
  ErrValue/1 -> Product2/1
  AssWaveErrAmpCoff/1 -> Product2/2
  Product2/1 -> Add2/1
  Ass_in/1 -> Switch4/3, Add2/2
  Switch4/1 -> Ass_out/1
  Add2/1 -> Switch4/1
  ErrSwitch/1 -> Switch4/2

== system GS_model/Subsystem2/Subsystem/Sensor/Ass/BodyAss(A&B&C&D)Model/Subsystem1/AssErrModel/AssErrSet/AssErrSet_WildValue ==
  Ass_in : Inport
  ErrValue : Inport  Port=2
  ErrSwitch : Inport  Port=3
  Add : Sum
  Switch2 : Switch  Criteria=u2 > Threshold  Threshold=0.5
  Ass_out : Outport
  wires:
  ErrValue/1 -> Add/1
  ErrSwitch/1 -> Switch2/2
  Switch2/1 -> Ass_out/1
  Ass_in/1 -> Switch2/3, Add/2
  Add/1 -> Switch2/1

== system GS_model/Subsystem2/Subsystem/Sensor/Ass/BodyAss(A&B&C&D)Model/Subsystem2/AssErrModel/AssErrSet/AssErrSet_Constant ==
  ErrSwitch : Inport
  Ass_in : Inport  Port=2
  Memory : Memory  InitialCondition=[0;0;0;0]
  Switch1 : Switch  Criteria=u2 > Threshold  Threshold=0.5
  Ass_out : Outport
  wires:
  Switch1/1 -> Ass_out/1, Memory/1
  Memory/1 -> Switch1/1
  Ass_in/1 -> Switch1/3
  ErrSwitch/1 -> Switch1/2

== system GS_model/Subsystem2/Subsystem/Sensor/Ass/BodyAss(A&B&C&D)Model/Subsystem2/AssErrModel/AssErrSet/AssErrSet_Jump ==
  Ass_in : Inport
  ErrValue : Inport  Port=2
  ErrSwitch : Inport  Port=3
  AssJumpErrAmpCoff : Inport  Port=4
  Add1 : Sum
  Product1 : Product  SaturateOnIntegerOverflow=on  OutDataTypeStr=Inherit: Same as first input
  Switch3 : Switch  Criteria=u2 > Threshold  Threshold=0.5
  Ass_out : Outport
  wires:
  Switch3/1 -> Ass_out/1
  ErrSwitch/1 -> Switch3/2
  Ass_in/1 -> Add1/2, Switch3/3
  AssJumpErrAmpCoff/1 -> Product1/2
  ErrValue/1 -> Product1/1
  Add1/1 -> Switch3/1
  Product1/1 -> Add1/1

== system GS_model/Subsystem2/Subsystem/Sensor/Ass/BodyAss(A&B&C&D)Model/Subsystem2/AssErrModel/AssErrSet/AssErrSet_Wave ==
  Ass_in : Inport
  ErrValue : Inport  Port=2
  ErrSwitch : Inport  Port=3
  AssWaveErrAmpCoff : Inport  Port=4
  Add2 : Sum
  Product2 : Product  SaturateOnIntegerOverflow=on  OutDataTypeStr=Inherit: Same as first input
  Switch4 : Switch  Criteria=u2 > Threshold  Threshold=0.5
  Ass_out : Outport
  wires:
  ErrSwitch/1 -> Switch4/2
  Add2/1 -> Switch4/1
  Switch4/1 -> Ass_out/1
  Ass_in/1 -> Add2/2, Switch4/3
  Product2/1 -> Add2/1
  AssWaveErrAmpCoff/1 -> Product2/2
  ErrValue/1 -> Product2/1

== system GS_model/Subsystem2/Subsystem/Sensor/Ass/BodyAss(A&B&C&D)Model/Subsystem2/AssErrModel/AssErrSet/AssErrSet_WildValue ==
  Ass_in : Inport
  ErrValue : Inport  Port=2
  ErrSwitch : Inport  Port=3
  Add : Sum
  Switch2 : Switch  Criteria=u2 > Threshold  Threshold=0.5
  Ass_out : Outport
  wires:
  Add/1 -> Switch2/1
  Ass_in/1 -> Add/2, Switch2/3
  Switch2/1 -> Ass_out/1
  ErrSwitch/1 -> Switch2/2
  ErrValue/1 -> Add/1

== system GS_model/Subsystem2/Subsystem/Sensor/Ass/BodyAss(A&B&C&D)Model/Subsystem3/AssErrModel/AssErrSet/AssErrSet_Constant ==
  ErrSwitch : Inport
  Ass_in : Inport  Port=2
  Memory : Memory  InitialCondition=[0;0;0;0]
  Switch1 : Switch  Criteria=u2 > Threshold  Threshold=0.5
  Ass_out : Outport
  wires:
  ErrSwitch/1 -> Switch1/2
  Ass_in/1 -> Switch1/3
  Memory/1 -> Switch1/1
  Switch1/1 -> Memory/1, Ass_out/1

== system GS_model/Subsystem2/Subsystem/Sensor/Ass/BodyAss(A&B&C&D)Model/Subsystem3/AssErrModel/AssErrSet/AssErrSet_Jump ==
  Ass_in : Inport
  ErrValue : Inport  Port=2
  ErrSwitch : Inport  Port=3
  AssJumpErrAmpCoff : Inport  Port=4
  Add1 : Sum
  Product1 : Product  SaturateOnIntegerOverflow=on  OutDataTypeStr=Inherit: Same as first input
  Switch3 : Switch  Criteria=u2 > Threshold  Threshold=0.5
  Ass_out : Outport
  wires:
  Product1/1 -> Add1/1
  Add1/1 -> Switch3/1
  ErrValue/1 -> Product1/1
  AssJumpErrAmpCoff/1 -> Product1/2
  Ass_in/1 -> Switch3/3, Add1/2
  ErrSwitch/1 -> Switch3/2
  Switch3/1 -> Ass_out/1

== system GS_model/Subsystem2/Subsystem/Sensor/Ass/BodyAss(A&B&C&D)Model/Subsystem3/AssErrModel/AssErrSet/AssErrSet_Wave ==
  Ass_in : Inport
  ErrValue : Inport  Port=2
  ErrSwitch : Inport  Port=3
  AssWaveErrAmpCoff : Inport  Port=4
  Add2 : Sum
  Product2 : Product  SaturateOnIntegerOverflow=on  OutDataTypeStr=Inherit: Same as first input
  Switch4 : Switch  Criteria=u2 > Threshold  Threshold=0.5
  Ass_out : Outport
  wires:
  ErrValue/1 -> Product2/1
  AssWaveErrAmpCoff/1 -> Product2/2
  Product2/1 -> Add2/1
  Ass_in/1 -> Switch4/3, Add2/2
  Switch4/1 -> Ass_out/1
  Add2/1 -> Switch4/1
  ErrSwitch/1 -> Switch4/2

== system GS_model/Subsystem2/Subsystem/Sensor/Ass/BodyAss(A&B&C&D)Model/Subsystem3/AssErrModel/AssErrSet/AssErrSet_WildValue ==
  Ass_in : Inport
  ErrValue : Inport  Port=2
  ErrSwitch : Inport  Port=3
  Add : Sum
  Switch2 : Switch  Criteria=u2 > Threshold  Threshold=0.5
  Ass_out : Outport
  wires:
  ErrValue/1 -> Add/1
  ErrSwitch/1 -> Switch2/2
  Switch2/1 -> Ass_out/1
  Ass_in/1 -> Switch2/3, Add/2
  Add/1 -> Switch2/1

== system GS_model/Subsystem2/Subsystem/Sensor/Ass/SolarPanelAss(E&F)Model/Subsystem/AssErrModel/AssErrSet/AssErrSet_Constant ==
  ErrSwitch : Inport
  Ass_in : Inport  Port=2
  Memory : Memory  InitialCondition=[0;0;0;0]
  Switch1 : Switch  Criteria=u2 > Threshold  Threshold=0.5
  Ass_out : Outport
  wires:
  Switch1/1 -> Ass_out/1, Memory/1
  Memory/1 -> Switch1/1
  Ass_in/1 -> Switch1/3
  ErrSwitch/1 -> Switch1/2

== system GS_model/Subsystem2/Subsystem/Sensor/Ass/SolarPanelAss(E&F)Model/Subsystem/AssErrModel/AssErrSet/AssErrSet_Jump ==
  Ass_in : Inport
  ErrValue : Inport  Port=2
  ErrSwitch : Inport  Port=3
  AssJumpErrAmpCoff : Inport  Port=4
  Add1 : Sum
  Product1 : Product  SaturateOnIntegerOverflow=on  OutDataTypeStr=Inherit: Same as first input
  Switch3 : Switch  Criteria=u2 > Threshold  Threshold=0.5
  Ass_out : Outport
  wires:
  Switch3/1 -> Ass_out/1
  ErrSwitch/1 -> Switch3/2
  Ass_in/1 -> Add1/2, Switch3/3
  AssJumpErrAmpCoff/1 -> Product1/2
  ErrValue/1 -> Product1/1
  Add1/1 -> Switch3/1
  Product1/1 -> Add1/1

== system GS_model/Subsystem2/Subsystem/Sensor/Ass/SolarPanelAss(E&F)Model/Subsystem/AssErrModel/AssErrSet/AssErrSet_Wave ==
  Ass_in : Inport
  ErrValue : Inport  Port=2
  ErrSwitch : Inport  Port=3
  AssWaveErrAmpCoff : Inport  Port=4
  Add2 : Sum
  Product2 : Product  SaturateOnIntegerOverflow=on  OutDataTypeStr=Inherit: Same as first input
  Switch4 : Switch  Criteria=u2 > Threshold  Threshold=0.5
  Ass_out : Outport
  wires:
  ErrSwitch/1 -> Switch4/2
  Add2/1 -> Switch4/1
  Switch4/1 -> Ass_out/1
  Ass_in/1 -> Add2/2, Switch4/3
  Product2/1 -> Add2/1
  AssWaveErrAmpCoff/1 -> Product2/2
  ErrValue/1 -> Product2/1

== system GS_model/Subsystem2/Subsystem/Sensor/Ass/SolarPanelAss(E&F)Model/Subsystem/AssErrModel/AssErrSet/AssErrSet_WildValue ==
  Ass_in : Inport
  ErrValue : Inport  Port=2
  ErrSwitch : Inport  Port=3
  Add : Sum
  Switch2 : Switch  Criteria=u2 > Threshold  Threshold=0.5
  Ass_out : Outport
  wires:
  Add/1 -> Switch2/1
  Ass_in/1 -> Add/2, Switch2/3
  Switch2/1 -> Ass_out/1
  ErrSwitch/1 -> Switch2/2
  ErrValue/1 -> Add/1

== system GS_model/Subsystem2/Subsystem/Sensor/Ass/SolarPanelAss(E&F)Model/Subsystem1/AssErrModel/AssErrSet/AssErrSet_Constant ==
  ErrSwitch : Inport
  Ass_in : Inport  Port=2
  Memory : Memory  InitialCondition=[0;0;0;0]
  Switch1 : Switch  Criteria=u2 > Threshold  Threshold=0.5
  Ass_out : Outport
  wires:
  Switch1/1 -> Ass_out/1, Memory/1
  Memory/1 -> Switch1/1
  Ass_in/1 -> Switch1/3
  ErrSwitch/1 -> Switch1/2

== system GS_model/Subsystem2/Subsystem/Sensor/Ass/SolarPanelAss(E&F)Model/Subsystem1/AssErrModel/AssErrSet/AssErrSet_Jump ==
  Ass_in : Inport
  ErrValue : Inport  Port=2
  ErrSwitch : Inport  Port=3
  AssJumpErrAmpCoff : Inport  Port=4
  Add1 : Sum
  Product1 : Product  SaturateOnIntegerOverflow=on  OutDataTypeStr=Inherit: Same as first input
  Switch3 : Switch  Criteria=u2 > Threshold  Threshold=0.5
  Ass_out : Outport
  wires:
  Switch3/1 -> Ass_out/1
  ErrSwitch/1 -> Switch3/2
  Ass_in/1 -> Add1/2, Switch3/3
  AssJumpErrAmpCoff/1 -> Product1/2
  ErrValue/1 -> Product1/1
  Add1/1 -> Switch3/1
  Product1/1 -> Add1/1

== system GS_model/Subsystem2/Subsystem/Sensor/Ass/SolarPanelAss(E&F)Model/Subsystem1/AssErrModel/AssErrSet/AssErrSet_Wave ==
  Ass_in : Inport
  ErrValue : Inport  Port=2
  ErrSwitch : Inport  Port=3
  AssWaveErrAmpCoff : Inport  Port=4
  Add2 : Sum
  Product2 : Product  SaturateOnIntegerOverflow=on  OutDataTypeStr=Inherit: Same as first input
  Switch4 : Switch  Criteria=u2 > Threshold  Threshold=0.5
  Ass_out : Outport
  wires:
  ErrSwitch/1 -> Switch4/2
  Add2/1 -> Switch4/1
  Switch4/1 -> Ass_out/1
  Ass_in/1 -> Add2/2, Switch4/3
  Product2/1 -> Add2/1
  AssWaveErrAmpCoff/1 -> Product2/2
  ErrValue/1 -> Product2/1

== system GS_model/Subsystem2/Subsystem/Sensor/Ass/SolarPanelAss(E&F)Model/Subsystem1/AssErrModel/AssErrSet/AssErrSet_WildValue ==
  Ass_in : Inport
  ErrValue : Inport  Port=2
  ErrSwitch : Inport  Port=3
  Add : Sum
  Switch2 : Switch  Criteria=u2 > Threshold  Threshold=0.5
  Ass_out : Outport
  wires:
  Add/1 -> Switch2/1
  Ass_in/1 -> Add/2, Switch2/3
  Switch2/1 -> Ass_out/1
  ErrSwitch/1 -> Switch2/2
  ErrValue/1 -> Add/1

== system GS_model/Subsystem2/Subsystem/Sensor/Gyro/GyroAModel/GyroErrSet/GyroErrSet/GyroErrSet_Constant/Triggered Subsystem1 ==
  In1 : Inport
  Enable : EnablePort
  Out1 : Outport
  wires:
  In1/1 -> Out1/1

== system GS_model/Subsystem2/Subsystem/Sensor/Gyro/GyroAModel/GyroErrSet/GyroErrSet/GyroErrSet_Constant/Triggered Subsystem2 ==
  In1 : Inport
  Enable : EnablePort
  Out1 : Outport
  wires:
  In1/1 -> Out1/1

== system GS_model/Subsystem2/Subsystem/Sensor/Gyro/GyroAModel/GyroErrSet/GyroErrSet/GyroErrSet_Constant/Triggered Subsystem8 ==
  In1 : Inport
  Enable : EnablePort
  Out1 : Outport
  wires:
  In1/1 -> Out1/1

== system GS_model/Subsystem2/Subsystem/Sensor/Gyro/GyroAModel/GyroErrSet/GyroErrSet/GyroErrSet_Jump/Triggered Subsystem1 ==
  In1 : Inport
  Enable : EnablePort
  Out1 : Outport
  wires:
  In1/1 -> Out1/1

== system GS_model/Subsystem2/Subsystem/Sensor/Gyro/GyroAModel/GyroErrSet/GyroErrSet/GyroErrSet_Jump/Triggered Subsystem2 ==
  In1 : Inport
  Enable : EnablePort
  Out1 : Outport
  wires:
  In1/1 -> Out1/1

== system GS_model/Subsystem2/Subsystem/Sensor/Gyro/GyroAModel/GyroErrSet/GyroErrSet/GyroErrSet_Jump/Triggered Subsystem8 ==
  In1 : Inport
  Enable : EnablePort
  Out1 : Outport
  wires:
  In1/1 -> Out1/1

== system GS_model/Subsystem2/Subsystem/Sensor/Gyro/GyroAModel/GyroErrSet/GyroErrSet/GyroErrSet_Wave/Triggered Subsystem1 ==
  In1 : Inport
  Enable : EnablePort
  Out1 : Outport
  wires:
  In1/1 -> Out1/1

== system GS_model/Subsystem2/Subsystem/Sensor/Gyro/GyroAModel/GyroErrSet/GyroErrSet/GyroErrSet_Wave/Triggered Subsystem2 ==
  In1 : Inport
  Enable : EnablePort
  Out1 : Outport
  wires:
  In1/1 -> Out1/1

== system GS_model/Subsystem2/Subsystem/Sensor/Gyro/GyroAModel/GyroErrSet/GyroErrSet/GyroErrSet_Wave/Triggered Subsystem8 ==
  In1 : Inport
  Enable : EnablePort
  Out1 : Outport
  wires:
  In1/1 -> Out1/1

== system GS_model/Subsystem2/Subsystem/Sensor/Gyro/GyroAModel/GyroErrSet/GyroErrSet/GyroErrSet_WildValue/Triggered Subsystem1 ==
  In1 : Inport
  Enable : EnablePort
  Out1 : Outport
  wires:
  In1/1 -> Out1/1

== system GS_model/Subsystem2/Subsystem/Sensor/Gyro/GyroAModel/GyroErrSet/GyroErrSet/GyroErrSet_WildValue/Triggered Subsystem2 ==
  In1 : Inport
  Enable : EnablePort
  Out1 : Outport
  wires:
  In1/1 -> Out1/1

== system GS_model/Subsystem2/Subsystem/Sensor/Gyro/GyroAModel/GyroErrSet/GyroErrSet/GyroErrSet_WildValue/Triggered Subsystem8 ==
  In1 : Inport
  Enable : EnablePort
  Out1 : Outport
  wires:
  In1/1 -> Out1/1

== system GS_model/Subsystem2/Subsystem/Sensor/Gyro/GyroBModel/GyroErrSet/GyroErrSet/GyroErrSet_Constant/Triggered Subsystem1 ==
  In1 : Inport
  Enable : EnablePort
  Out1 : Outport
  wires:
  In1/1 -> Out1/1

== system GS_model/Subsystem2/Subsystem/Sensor/Gyro/GyroBModel/GyroErrSet/GyroErrSet/GyroErrSet_Constant/Triggered Subsystem2 ==
  In1 : Inport
  Enable : EnablePort
  Out1 : Outport
  wires:
  In1/1 -> Out1/1

== system GS_model/Subsystem2/Subsystem/Sensor/Gyro/GyroBModel/GyroErrSet/GyroErrSet/GyroErrSet_Constant/Triggered Subsystem8 ==
  In1 : Inport
  Enable : EnablePort
  Out1 : Outport
  wires:
  In1/1 -> Out1/1

== system GS_model/Subsystem2/Subsystem/Sensor/Gyro/GyroBModel/GyroErrSet/GyroErrSet/GyroErrSet_Jump/Triggered Subsystem1 ==
  In1 : Inport
  Enable : EnablePort
  Out1 : Outport
  wires:
  In1/1 -> Out1/1

== system GS_model/Subsystem2/Subsystem/Sensor/Gyro/GyroBModel/GyroErrSet/GyroErrSet/GyroErrSet_Jump/Triggered Subsystem2 ==
  In1 : Inport
  Enable : EnablePort
  Out1 : Outport
  wires:
  In1/1 -> Out1/1
